simulink model "lab2"  (R2023b)
settings: Solver=ode113  StartTime=0.0  StopTime=10.0  RelTol=1e-10
values from neighbouring files (symbols this model uses):
  A = 2    [lab21.m]
  B = 8    [lab21.m]
  C = 3    [lab21.m]
  D = 9    [lab21.m]
  g = 9.81    [lab0.m]
  Kd = [100,0 ... (first row only)    [dane2nh.m]    (also in danenh.m = [1000,0; lab21.m = [D11,D12)
  Kp = [P11,P12 ... (first row only)    [lab21.m]
  theta1 = 3.1    [lab0.m]
  theta2 = 9.5    [lab0.m]
  theta3 = 0.24    [lab0.m]
  theta4 = 0.77    [lab0.m]
settings Model: Creator=alozins2  LastModifiedBy=alozins2

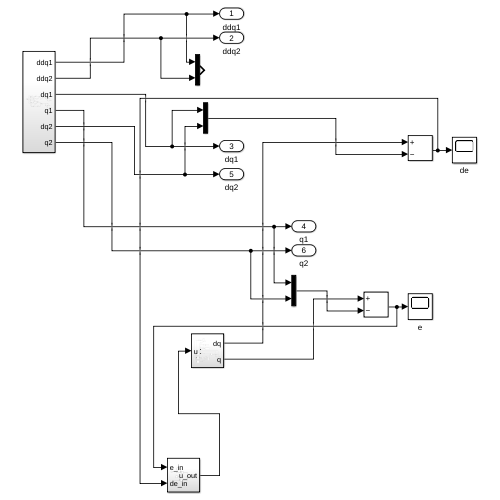
[thumbnail: Simulink's stored preview of the top-level diagram]
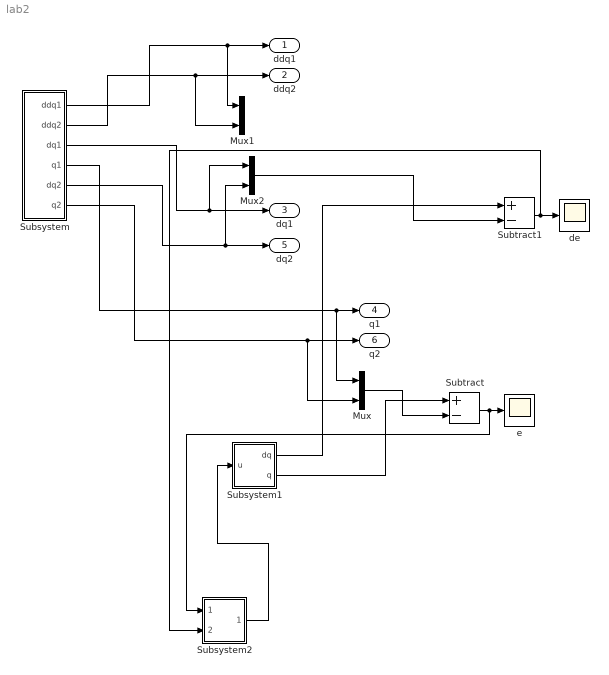
== system lab2 ==
  Mux : Mux  Inputs=2
  Mux1 : Mux  Inputs=2
  Mux2 : Mux  Inputs=2
  Subsystem : Subsystem
  Subsystem1 : Subsystem
  Subsystem2 : Subsystem
  Subtract : Sum  Inputs=+-
  Subtract1 : Sum  Inputs=+-
  de : Scope
  e : Scope
  ddq1 : Outport
  ddq2 : Outport  Port=2
  dq1 : Outport  Port=3
  q1 : Outport  Port=4
  dq2 : Outport  Port=5
  q2 : Outport  Port=6
  wires:
  Subsystem/1(ddq1) -> Mux1/1, ddq1/1
  Subsystem/2(ddq2) -> Mux1/2, ddq2/1
  Subsystem/4(q1) -> Mux/1, q1/1
  Subsystem/5(dq2) -> dq2/1, Mux2/2
  Subsystem/6(q2) -> Mux/2, q2/1
  Subsystem/3(dq1) -> Mux2/1, dq1/1
  Mux/1 -> Subtract/2
  Subsystem1/2(q) -> Subtract/1
  Subtract/1 -> Subsystem2/1(e_in), e/1
  Subtract1/1 -> Subsystem2/2(de_in), de/1
  Subsystem1/1(dq) -> Subtract1/1
  Mux2/1 -> Subtract1/2
  Subsystem2/1(u_out) -> Subsystem1/1(u)

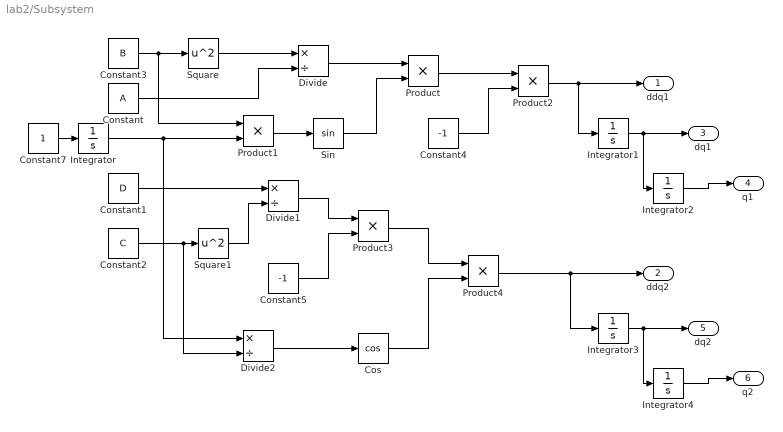
== system lab2/Subsystem ==
  Constant : Constant  Value=A
  Constant1 : Constant  Value=D
  Constant2 : Constant  Value=C
  Constant3 : Constant  Value=B
  Constant4 : Constant  Value=-1
  Constant5 : Constant  Value=-1
  Constant7 : Constant
  Cos : Trigonometry  Operator=cos
  Divide : Product  Inputs=*/
  Divide1 : Product  Inputs=*/
  Divide2 : Product  Inputs=*/
  Integrator : Integrator
  Integrator1 : Integrator  InitialCondition=B/A
  Integrator2 : Integrator
  Integrator3 : Integrator
  Integrator4 : Integrator  InitialCondition=D
  Product{,1..4} (5 alike) : Product
  Sin : Trigonometry
  Square : Math  Operator=square
  Square1 : Math  Operator=square
  ddq1 : Outport
  ddq2 : Outport  Port=2
  dq1 : Outport  Port=3
  q1 : Outport  Port=4
  dq2 : Outport  Port=5
  q2 : Outport  Port=6
  wires:
  Constant/1 -> Divide/2
  Divide1/1 -> Product3/1
  Divide/1 -> Product/1
  Product3/1 -> Product4/1
  Square1/1 -> Divide1/2
  Constant2/1 -> Divide2/2, Square1/1
  Integrator1/1 -> dq1/1, Integrator2/1
  Product2/1 -> ddq1/1, Integrator1/1
  Product/1 -> Product2/1
  Constant5/1 -> Product3/2
  Integrator2/1 -> q1/1
  Cos/1 -> Product4/2
  Square/1 -> Divide/1
  Constant4/1 -> Product2/2
  Integrator/1 -> Divide2/1, Product1/2
  Integrator4/1 -> q2/1
  Divide2/1 -> Cos/1
  Integrator3/1 -> dq2/1, Integrator4/1
  Sin/1 -> Product/2
  Product1/1 -> Sin/1
  Product4/1 -> ddq2/1, Integrator3/1
  Constant3/1 -> Product1/1, Square/1
  Constant7/1 -> Integrator/1
  Constant1/1 -> Divide1/1

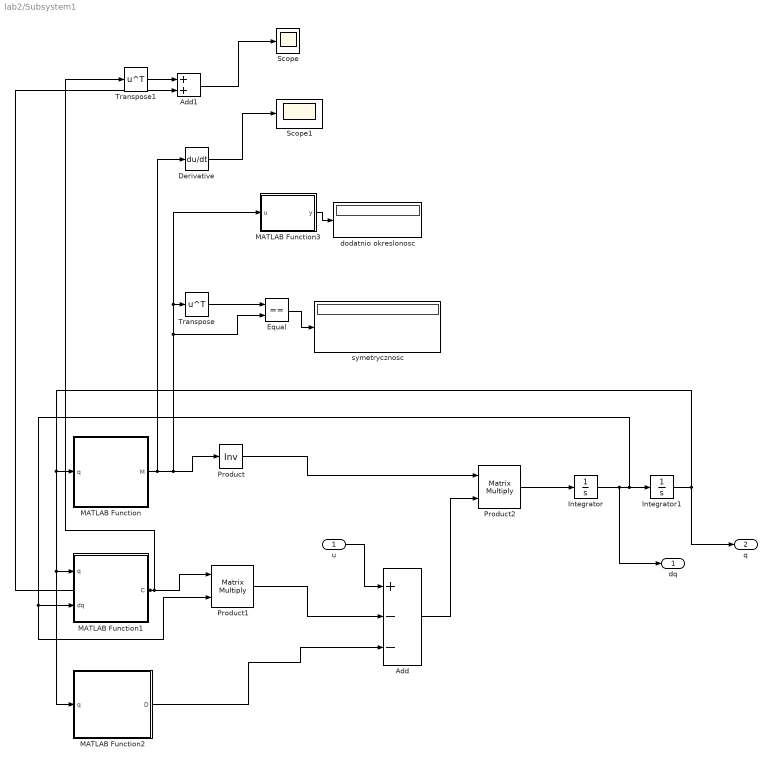
== system lab2/Subsystem1 ==
  u : Inport
  Add : Sum  Inputs=+--
  Add1 : Sum
  Derivative : Derivative
  Equal : RelationalOperator  Operator===  OutDataTypeStr=boolean  RndMeth=Simplest  InputSameDT=off
  Integrator : Integrator  InitialCondition=[0;0]
  Integrator1 : Integrator  InitialCondition=[-3.14/2;0]
  MATLAB Function : MATLAB Function  TreatAsAtomicUnit=on
  MATLAB Function1 : MATLAB Function  TreatAsAtomicUnit=on
  MATLAB Function2 : MATLAB Function  TreatAsAtomicUnit=on
  MATLAB Function3 : MATLAB Function  TreatAsAtomicUnit=on
  Product : Product  Inputs=/  Multiplication=Matrix(*)
  Product1 : Product  Multiplication=Matrix(*)
  Product2 : Product  Multiplication=Matrix(*)
  Scope : Scope
  Scope1 : Scope
  Transpose : Math  Operator=transpose
  Transpose1 : Math  Operator=transpose
  dodatnio okreslonosc : Display
  symetrycznosc : Display
  dq : Outport
  q : Outport  Port=2
  wires:
  MATLAB Function2/1(D) -> Add/3
  Product1/1 -> Add/2
  MATLAB Function/1(M) -> Derivative/1, Equal/2, MATLAB Function3/1(u), Transpose/1, Product/1
  Product2/1 -> Integrator/1
  MATLAB Function1/1(C) -> Product1/1, Transpose1/1, Add1/2
  Integrator/1 -> dq/1, Product1/2, MATLAB Function1/2(dq), Integrator1/1
  Product/1 -> Product2/1
  u/1 -> Add/1
  Add/1 -> Product2/2
  Integrator1/1 -> q/1, MATLAB Function2/1(q), MATLAB Function1/1(q), MATLAB Function/1(q)
  Transpose/1 -> Equal/1
  Equal/1 -> symetrycznosc/1
  MATLAB Function3/1(y) -> dodatnio okreslonosc/1
  Transpose1/1 -> Add1/1
  Add1/1 -> Scope/1
  Derivative/1 -> Scope1/1

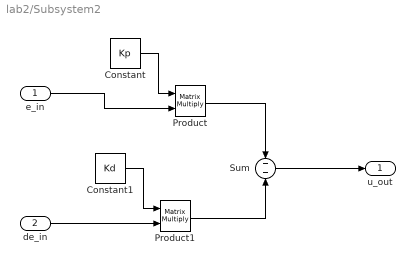
== system lab2/Subsystem2 ==
  e_in : Inport
  de_in : Inport  Port=2
  Constant : Constant  Value=Kp
  Constant1 : Constant  Value=Kd
  Product : Product  Multiplication=Matrix(*)
  Product1 : Product  Multiplication=Matrix(*)
  Sum : Sum  Inputs=--
  u_out : Outport
  wires:
  de_in/1 -> Product1/2
  Product/1 -> Sum/1
  Product1/1 -> Sum/2
  Constant/1 -> Product/1
  Constant1/1 -> Product1/1
  e_in/1 -> Product/2
  Sum/1 -> u_out/1

== matlab function lab2/Subsystem1/MATLAB Function1 ==
  data: q input; dq input; C output; theta1 parameter; theta3 parameter; theta4 parameter
function C = Corliolis(q,dq,theta1, theta3, theta4)

q1=q(1);
q2=q(2);

dq1=dq(1);
dq2=dq(2);

C=[-dq2, -(dq1+dq2);
    dq1,0]*0.3*theta4*sin(q2);

== matlab function lab2/Subsystem1/MATLAB Function ==
  data: q input; M output; theta1 parameter; theta3 parameter; theta4 parameter
function M = interiaMatrix(q,theta1, theta3, theta4)

q1=q(1);
q2=q(2);

M=[theta1 + 0.6*theta4*cos(q2), theta3 + 0.3*theta4*cos(q2);
    theta3 + 0.3*theta4*cos(q2), theta3];

== matlab function lab2/Subsystem1/MATLAB Function2 ==
  data: q input; D output; g parameter; theta2 parameter; theta4 parameter
function D = Gravity(q,g,theta2,theta4)

q1=q(1);
q2=q(2);

D=g*[theta2*cos(q1) + theta4*cos(q1+q2);
    theta4*cos(q1+q2)];

== matlab function lab2/Subsystem1/MATLAB Function3 ==
  data: u input; y output
function y = fcn(u)

y = det(u);
